simulink model "EV_template"  (R2024b)
settings: Solver=ode45  StartTime=SIM.t_min  StopTime=SIM.t_simul  FixedStep=1e-2  MaxStep=1e-3  RelTol=1e-3  EnableMultiTasking=on
InitFcn:
  | init_ev
undefined symbols (not defined in the file or in its folder): BATp, CHAp, CYCL, RDp
libraries: simulink x1
settings Model: Creator=Tony  LastModifiedBy=philippe.barrade
settings SolverCC: ZeroCrossAlgorithm=Non-adaptive  AlgebraicLoopSolver=TrustRegion
settings DataIOCC: SaveFormat=Array  SignalLoggingSaveFormat=ModelDataLogs  ReturnWorkspaceOutputs=off  SignalLoggingName=sigsOut
settings OptimizationCC: BooleanDataType=off  ExpressionDepthLimit=2147483647  LifeSpan=inf
settings DebuggingCC: SaveWithParameterizedLinksMsg=none  UnderspecifiedInitializationDetection=Classic  MergeDetectMultiDrivingBlocksExec=none  SignalResolutionControl=TryResolveAllWithWarning  MultiTaskDSMMsg=warning  MultiTaskCondExecSysMsg=none  FcnCallInpInsideContextMsg=warning  UnconnectedInputMsg=warning  UnconnectedOutputMsg=warning  UnconnectedLineMsg=warning  StateNameClashWarn=warning  SFUnexpectedBacktrackingDiag=warning  SFNoUnconditionalDefaultTransitionDiag=warning  ArithmeticOperatorsInVariantConditions=warning
settings HardwareCC: ProdBitPerPointer=32  ProdBitPerSizeT=32  ProdBitPerPtrDiffT=32  ProdLargestAtomicFloat=None  ProdIntDivRoundTo=Undefined  ProdEndianess=Unspecified  ProdWordSize=32  ProdHWDeviceType=32-bit Generic  TargetUnknown=on
settings ModelReferenceCC: EnableRefExpFcnMdlSchedulingChecks=on  PropagateSignalLabelsOutOfModel=off
settings SFSimCC: CustomCodeUndefinedFunction=UseInterfaceOnly
settings RTWCC: GPUComputeCapability=3.5
settings CodeAppCC: StateflowObjectComments=on
settings GRTTargetCC: TargetLangStandard=C89/C90 (ANSI)  CombineOutputUpdateFcns=off  GRTInterface=on
settings ConfigComp: CovMetricSettings=dw  CovSaveCumulativeToWorkspaceVar=on  CovSaveSingleToWorkspaceVar=on

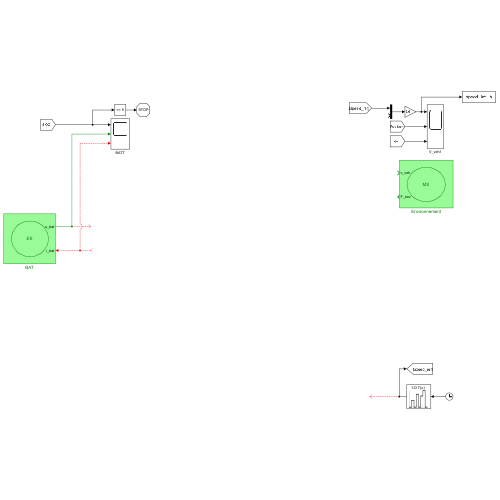
[thumbnail: Simulink's stored preview of the top-level diagram]
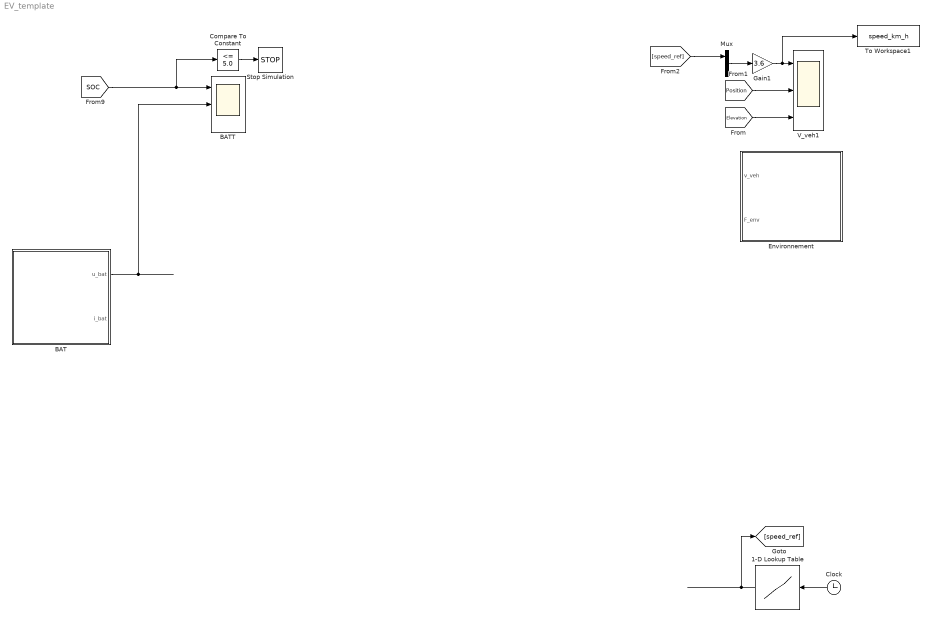
== system EV_template ==
  1-D Lookup Table : Lookup_n-D  NumberOfTableDimensions=1  BreakpointsForDimension1=CYCL.time  Table=CYCL.speed  InternalRulePriority=Speed  RndMeth=Simplest
  BAT : Subsystem
      settings: PortSchema="{\"entries\":[{\"content\":{\"sides\":[{\"content\":{\"connectorIds\":[]},\"type\":\"ConnectorPlacement.EquallySpacedRectSide\",\"uuid\":\"f966fbbf-87fd-4eae-ac75-d366ea856ba9\"},{\"content\":{\"connectorIds\":[\"Out1\",\"In1\"],\"side\":\"RIGHT\"},\"type\":\"ConnectorPlacement.EquallySpacedRectSide\",\"uuid\":\"019a522f-a65b-4de4-928a-6ec503aa07e1\"},{\"content\":{\"connectorIds\":[],\"side\":\"TOP\"},\"type\":\"ConnectorPlacement.EquallySpacedRectSide\",\"uuid\":\"2e7350c2-17d6-436e-acd0-d7bc7ebcdc21\"}]},\"type\":\"ConnectorPlacement.EquallySpacedConnector\",\"uuid\":\"cf36ffa8-c853-4b91-8b40-e4ddcf06bdb1\"}],\"packageUris\":[\"http://schema.mathworks.com/mf0/Connector/R2020b\"],\"version\":\"1.0\"}"
      mask Display:
      | plot(0,0,100,100, 1.2*[50,57.68,60.77,63.08,64.97,66.58,68,69.26,70.4, 	71.42,72.36,78.28,80,78.28,72.36,71.42,70.4, 	69.26,68,66.58,64.97,63.08,60.77,57.68,50,42.32, 	39.23,36.92,35.03,33.42,32,30.74,29.6,28.58, 	27.64,21.72,20,21.72,27.64,28.58,29.6,30.74,32, 	33.42,35.03,36.92,39.23,42.32,50]-10, 1.2*[20,21,22,23,24,25,26,27,28,29,30,40,50,60,70,71,72, 	73,74,75,76,77,78,79,80,79,78,77,76,75,74,73,72, 	71,70,60,50,40,30,29,28,27,26,25,24,23,22,21,20]-10)
      | disp('ES')
  BATT : Scope  NumInputPorts=3
  Clock : Clock
  Compare To Constant : simulink/Logic and Bit Operations/Compare To Constant  relop=<=  const=5.0  OutDataTypeStr=boolean
  Environnement : Subsystem
      settings: PortSchema="{\"entries\":[{\"content\":{\"sides\":[{\"content\":{\"connectorIds\":[\"In1\",\"Out1\"]},\"type\":\"ConnectorPlacement.EquallySpacedRectSide\",\"uuid\":\"f966fbbf-87fd-4eae-ac75-d366ea856ba9\"},{\"content\":{\"connectorIds\":[],\"side\":\"RIGHT\"},\"type\":\"ConnectorPlacement.EquallySpacedRectSide\",\"uuid\":\"019a522f-a65b-4de4-928a-6ec503aa07e1\"},{\"content\":{\"connectorIds\":[],\"side\":\"TOP\"},\"type\":\"ConnectorPlacement.EquallySpacedRectSide\",\"uuid\":\"2e7350c2-17d6-436e-acd0-d7bc7ebcdc21\"}]},\"type\":\"ConnectorPlacement.EquallySpacedConnector\",\"uuid\":\"cf36ffa8-c853-4b91-8b40-e4ddcf06bdb1\"}],\"packageUris\":[\"http://schema.mathworks.com/mf0/Connector/R2020b\"],\"version\":\"1.0\"}"
      mask Display:
      | plot(0,0,100,100, 1.2*[50,57.68,60.77,63.08,64.97,66.58,68,69.26,70.4, 	71.42,72.36,78.28,80,78.28,72.36,71.42,70.4, 	69.26,68,66.58,64.97,63.08,60.77,57.68,50,42.32, 	39.23,36.92,35.03,33.42,32,30.74,29.6,28.58, 	27.64,21.72,20,21.72,27.64,28.58,29.6,30.74,32, 	33.42,35.03,36.92,39.23,42.32,50]-10, 1.2*[20,21,22,23,24,25,26,27,28,29,30,40,50,60,70,71,72, 	73,74,75,76,77,78,79,80,79,78,77,76,75,74,73,72, 	71,70,60,50,40,30,29,28,27,26,25,24,23,22,21,20]-10)
      | disp('MS')
  Gain1 : Gain  Gain=3.6
  Mux : Mux  Inputs=2
  Stop Simulation : Stop
  To Workspace1 : ToWorkspace  VariableName=speed_km_h  SampleTime=-1
  V_veh1 : Scope  NumInputPorts=3
  wires:
  BAT/1(u_bat) -> BATT/2
  [SOC] -> Compare To Constant/1, BATT/1
  ? -> BAT/1(i_bat), BATT/3
  [Position] -> V_veh1/2
  [Elevation] -> V_veh1/3
  Gain1/1 -> To Workspace1/1, V_veh1/1
  Mux/1 -> Gain1/1
  1-D Lookup Table/1 -> [speed_ref]
  [speed_ref] -> Mux/1
  Compare To Constant/1 -> Stop Simulation/1
  Clock/1 -> 1-D Lookup Table/1

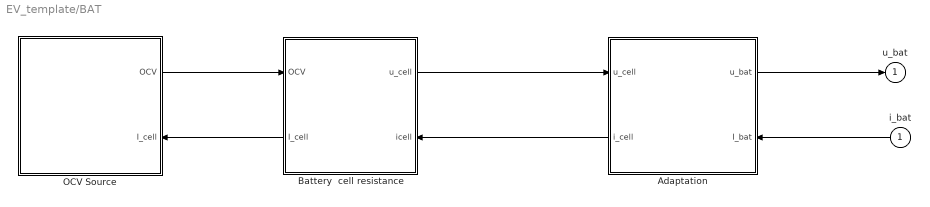
== system EV_template/BAT ==
  i_bat : Inport
  Adaptation : Subsystem  mask(CM){}
      settings: PortSchema="{\"entries\":[{\"content\":{\"sides\":[{\"content\":{\"connectorIds\":[\"In1\",\"Out2\"]},\"type\":\"ConnectorPlacement.EquallySpacedRectSide\",\"uuid\":\"43b53794-c784-4d35-8a91-f1490638489e\"},{\"content\":{\"connectorIds\":[\"Out1\",\"In2\"],\"side\":\"RIGHT\"},\"type\":\"ConnectorPlacement.EquallySpacedRectSide\",\"uuid\":\"00b1a1a6-7269-4083-abb9-f1208d9f3b4c\"},{\"content\":{\"connectorIds\":[],\"side\":\"TOP\"},\"type\":\"ConnectorPlacement.EquallySpacedRectSide\",\"uuid\":\"3919f87a-9a68-4334-b84e-5fe8c9917a96\"}]},\"type\":\"ConnectorPlacement.EquallySpacedConnector\",\"uuid\":\"9597a696-d499-48cc-bc44-63d792d74754\"}],\"packageUris\":[\"http://schema.mathworks.com/mf0/Connector/R2020b\"],\"version\":\"1.0\"}"
      mask Display: plot(0,0,100,100, [10,10,90,90,10],[90,10,10,90,90], [90,10,90],[10,50,90])
  Battery  cell resistance : Subsystem  mask(Hacheur){}
      settings: PortSchema="{\"entries\":[{\"content\":{\"sides\":[{\"content\":{\"connectorIds\":[\"In1\",\"Out2\"]},\"type\":\"ConnectorPlacement.EquallySpacedRectSide\",\"uuid\":\"43b53794-c784-4d35-8a91-f1490638489e\"},{\"content\":{\"connectorIds\":[\"Out1\",\"In2\"],\"side\":\"RIGHT\"},\"type\":\"ConnectorPlacement.EquallySpacedRectSide\",\"uuid\":\"00b1a1a6-7269-4083-abb9-f1208d9f3b4c\"},{\"content\":{\"connectorIds\":[],\"side\":\"TOP\"},\"type\":\"ConnectorPlacement.EquallySpacedRectSide\",\"uuid\":\"3919f87a-9a68-4334-b84e-5fe8c9917a96\"}]},\"type\":\"ConnectorPlacement.EquallySpacedConnector\",\"uuid\":\"9597a696-d499-48cc-bc44-63d792d74754\"}],\"packageUris\":[\"http://schema.mathworks.com/mf0/Connector/R2020b\"],\"version\":\"1.0\"}"
      mask Display: plot(0,0,100,100,[10,10,90,90,10],[90,10,10,90,90])
  OCV Source : Subsystem
      settings: PortSchema="{\"entries\":[{\"content\":{\"sides\":[{\"content\":{\"connectorIds\":[]},\"type\":\"ConnectorPlacement.EquallySpacedRectSide\",\"uuid\":\"87b7c904-bcc3-4a98-87e1-6b58a76e8897\"},{\"content\":{\"connectorIds\":[\"Out1\",\"In1\"],\"side\":\"RIGHT\"},\"type\":\"ConnectorPlacement.EquallySpacedRectSide\",\"uuid\":\"67c0e4e9-ec6a-4f26-b099-e0fb0eaa0b35\"},{\"content\":{\"connectorIds\":[],\"side\":\"TOP\"},\"type\":\"ConnectorPlacement.EquallySpacedRectSide\",\"uuid\":\"8fb5181e-f6b7-4828-b0d6-b00809980f9d\"}]},\"type\":\"ConnectorPlacement.EquallySpacedConnector\",\"uuid\":\"ac4387ff-8ed1-4b4c-b503-b7c8237b5a9a\"}],\"packageUris\":[\"http://schema.mathworks.com/mf0/Connector/R2020b\"],\"version\":\"1.0\"}"
      mask Display:
      | plot(0,0,100,100, 1.2*[50,57.68,60.77,63.08,64.97,66.58,68,69.26,70.4, 	71.42,72.36,78.28,80,78.28,72.36,71.42,70.4, 	69.26,68,66.58,64.97,63.08,60.77,57.68,50,42.32, 	39.23,36.92,35.03,33.42,32,30.74,29.6,28.58, 	27.64,21.72,20,21.72,27.64,28.58,29.6,30.74,32, 	33.42,35.03,36.92,39.23,42.32,50]-10, 1.2*[20,21,22,23,24,25,26,27,28,29,30,40,50,60,70,71,72, 	73,74,75,76,77,78,79,80,79,78,77,76,75,74,73,72, 	71,70,60,50,40,30,29,28,27,26,25,24,23,22,21,20]-10)
      | disp('MS')
  u_bat : Outport  InitialOutput=0
  wires:
  Adaptation/1(u_bat) -> u_bat/1
  i_bat/1 -> Adaptation/2(I_bat)
  Adaptation/2(i_cell) -> Battery  cell resistance/2(icell)
  Battery  cell resistance/1(u_cell) -> Adaptation/1(u_cell)
  OCV Source/1(OCV) -> Battery  cell resistance/1(OCV)
  Battery  cell resistance/2(I_cell) -> OCV Source/1("I_cell ")

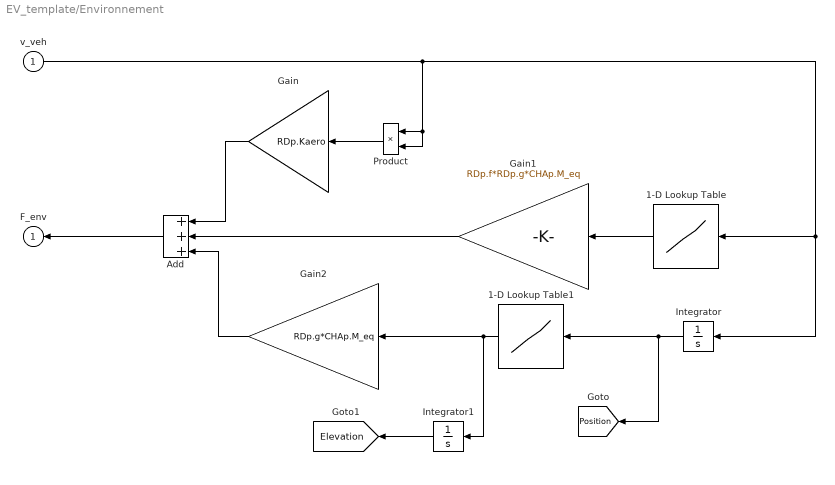
== system EV_template/Environnement ==
  v_veh : Inport
  1-D Lookup Table : Lookup_n-D  NumberOfTableDimensions=1  BreakpointsForDimension1=[-100 -1 0 1 100]  Table=[-1 -1 0 1 1]  InternalRulePriority=Speed  RndMeth=Simplest
  1-D Lookup Table1 : Lookup_n-D  NumberOfTableDimensions=1  BreakpointsForDimension1=CYCL.position  Table=CYCL.slope  InternalRulePriority=Speed  RndMeth=Simplest
  Add : Sum  Inputs=+++
  Gain : Gain  Gain=RDp.Kaero  SaturateOnIntegerOverflow=on  OutDataTypeStr=Inherit: Same as input  ParamDataTypeStr=Inherit: Same as input
  Gain1 : Gain  Gain=RDp.f*RDp.g*CHAp.M_eq  SaturateOnIntegerOverflow=on  OutDataTypeStr=Inherit: Same as input  ParamDataTypeStr=Inherit: Same as input
  Gain2 : Gain  Gain=RDp.g*CHAp.M_eq  SaturateOnIntegerOverflow=on  OutDataTypeStr=Inherit: Same as input  ParamDataTypeStr=Inherit: Same as input
  Integrator : Integrator
  Integrator1 : Integrator
  Product : Product  InputSameDT=on  SaturateOnIntegerOverflow=on  OutDataTypeStr=Inherit: Same as first input
  F_env : Outport  InitialOutput=0
  tag scope: Elevation=global, Position=global
  wires:
  Product/1 -> Gain/1
  Add/1 -> F_env/1
  v_veh/1 -> Product/1, Product/2, Integrator/1, 1-D Lookup Table/1
  Gain/1 -> Add/1
  Gain1/1 -> Add/2
  1-D Lookup Table/1 -> Gain1/1
  Integrator/1 -> 1-D Lookup Table1/1, [Position]
  1-D Lookup Table1/1 -> Gain2/1, Integrator1/1
  Gain2/1 -> Add/3
  Integrator1/1 -> [Elevation]

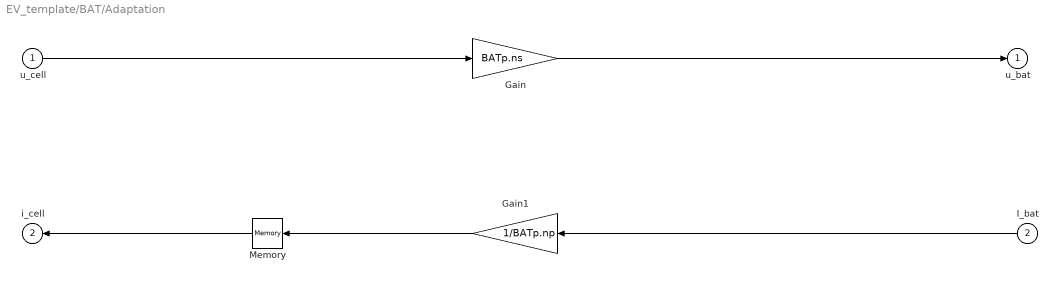
== system EV_template/BAT/Adaptation ==
  u_cell : Inport
  I_bat : Inport  Port=2
  Gain : Gain  Gain=BATp.ns
  Gain1 : Gain  Gain=1/BATp.np
  Memory : Memory
  u_bat : Outport  InitialOutput=0
  i_cell : Outport  Port=2  InitialOutput=0
  wires:
  Gain/1 -> u_bat/1
  I_bat/1 -> Gain1/1
  u_cell/1 -> Gain/1
  Gain1/1 -> Memory/1
  Memory/1 -> i_cell/1

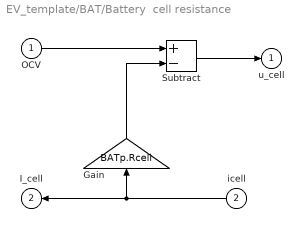
== system EV_template/BAT/Battery  cell resistance ==
  OCV : Inport
  icell : Inport  Port=2
  Gain : Gain  Gain=BATp.Rcell
  Subtract : Sum  Inputs=+-
  u_cell : Outport  InitialOutput=0
  I_cell : Outport  Port=2  InitialOutput=0
  wires:
  Subtract/1 -> u_cell/1
  icell/1 -> I_cell/1, Gain/1
  Gain/1 -> Subtract/2
  OCV/1 -> Subtract/1

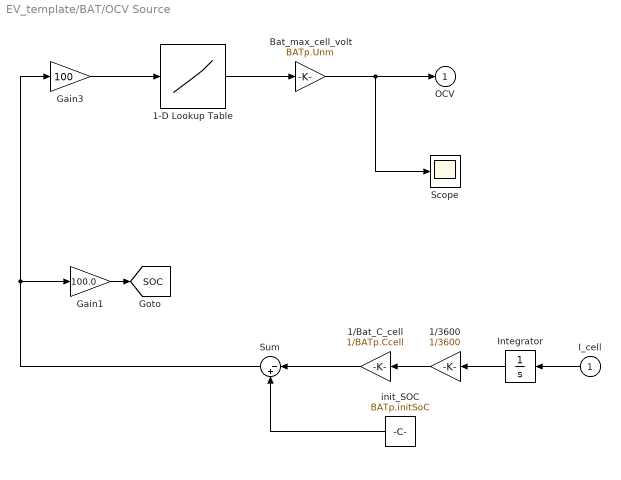
== system EV_template/BAT/OCV Source ==
  "I_cell " : Inport
  1-D Lookup Table : Lookup_n-D  NumberOfTableDimensions=1  BreakpointsForDimension1=BATp.SoC  Table=BATp.OCV  InternalRulePriority=Speed  RndMeth=Simplest
  1/3600 : Gain  Gain=1/3600
  1/Bat_C_cell : Gain  Gain=1/BATp.Ccell
  Bat_max_cell_volt : Gain  Gain=BATp.Unm
  Gain1 : Gain  Gain=100.0
  Gain3 : Gain  Gain=100
  Integrator : Integrator
  Scope : Scope
  Sum : Sum  Inputs=|-+
  init_SOC : Constant  Value=BATp.initSoC
  OCV : Outport  InitialOutput=0
  tag scope: SOC=global
  wires:
  Sum/1 -> Gain1/1, Gain3/1
  1-D Lookup Table/1 -> Bat_max_cell_volt/1
  Gain3/1 -> 1-D Lookup Table/1
  Integrator/1 -> 1/3600/1
  init_SOC/1 -> Sum/2
  1/Bat_C_cell/1 -> Sum/1
  "I_cell "/1 -> Integrator/1
  1/3600/1 -> 1/Bat_C_cell/1
  Bat_max_cell_volt/1 -> Scope/1, OCV/1
  Gain1/1 -> [SOC]
